simulink model "Mission__SimulatorModel"  (Simulink 10.1)
settings: Solver=ode8  StartTime=0.0  StopTime=100000  FixedStep=time_step  RelTol=1e-3
StartFcn:
  | % copyfile(char(CurrentFolder + "\3DModels\" + string(MODELO_3D)), char(CurrentFolder + "\" + string(MODELO_3D)));
StopFcn:
  | % delete(MODELO_3D)
values from neighbouring files (symbols this model uses):
  Aileron_Trim = -deltaa_trim_med/2    [Trim_ArcDME2.m]
  Elevator_Trim = deltae_trim_med    [Trim_ArcDME2.m]    (also in Trim_ClimbXZ2.m; Trim_CruiseThetaXZ2.m)
  Engine_Trim = lever_trim_med    [Trim_ArcDME2.m]    (also in Trim_ClimbXZ2.m; Trim_CruiseThetaXZ2.m)
  phi_ini = phi_ini_trim_med    [Trim_ArcDME2.m]
  u_ini = u_ini_trim_med    [Trim_ArcDME2.m]    (also in Trim_ClimbXZ2.m; Trim_CruiseThetaXZ2.m)
  v_ini = v_ini_trim2    [Trim_ArcDME2.m]    (also in Trim_ClimbXZ2.m; Trim_CruiseThetaXZ2.m)
  w_ini = -UVW_aux(3)    [Trim_ArcDME2.m]    (also in Trim_ClimbXZ2.m = -UVW_aux2(3) + UVW_aux1(3); Trim_CruiseThetaXZ2.m)
undefined symbols (not defined in the file or in its folder): AoA_alpha_max, AoA_beta_max, b, c, cargo_mass, CD0_interp, CD_ajus_coef, CD_beta_interp, CD_mach_reg, CDde, CDflap, CDgear, CDi, CDsb, CDsp, CL_ajus_coef, CL_alpha_interp, CL_alpha_reg, Clb, Clda_interp, CLde, Cldr, Clp, Clr, Cm0, Cm_alpha, Cmadot, Cmde_ajus_coef, Cmde_interp, Cmq, Cnb, Cndr, Cnr, Coef_Aileron_Beta, Coef_Aileron_Phi, Coef_Aileron_Rudder, Coef_Elevator_Alpha, Coef_Rudder_Aileron, Coef_Rudder_Beta, CYb, dCLflap, dfuel, dfuel0, e0_0, e1_0, e2_0, e3_0, fuel, fuel_density, fuel_max, g, GeoDate_Ap, GeoDate_Day, GeoDate_LatLongElv, GeoDate_Time, Ixx, Ixz, Iyy, Izz, kCDge_interp ... (+35)
libraries: aerolibconvert2 x17, aerolibutil x14, dsppolyfun x7, aerolibactuator x5, sharedtransform x4, robotcorelib x4, simulink x3, visionstatistics x3, vrlib x2, aerolibasang x1
(part 3 of 3)

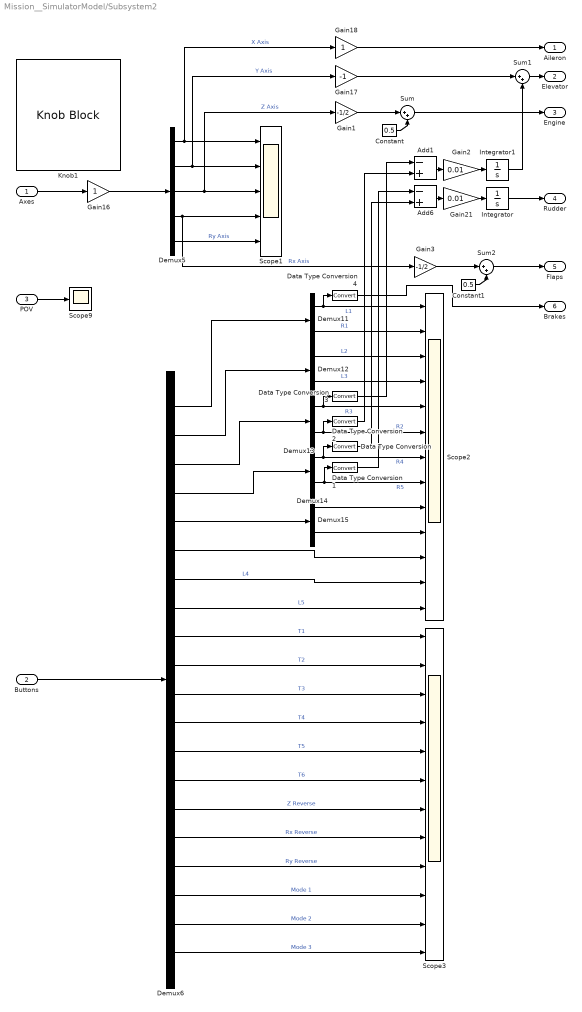
== system Mission__SimulatorModel/Subsystem2 ==
  Axes : Inport
  Buttons : Inport  Port=2
  POV : Inport  Port=3
  Add1 : Sum  Inputs=-+
  Add6 : Sum  Inputs=-+
  Constant : Constant  Value=0.5
  Constant1 : Constant  Value=0.5
  Data Type Conversion{,1..4} (5 alike) : DataTypeConversion
  Demux{11..15} (5 alike) : Demux  Outputs=2
  Demux5 : Demux  Outputs=5
  Demux6 : Demux  Outputs=20
  Gain1 : Gain  Gain=-1/2
  Gain16 : Gain
  Gain17 : Gain  Gain=-1
  Gain18 : Gain
  Gain2 : Gain  Gain=0.01
  Gain21 : Gain  Gain=0.01
  Gain3 : Gain  Gain=-1/2
  Integrator : Integrator  LowerSaturationLimit=inf
  Integrator1 : Integrator  LowerSaturationLimit=inf
  Knob1 : KnobBlock  LabelPosition=Hide  ScaleMax=1
  Scope1 : Scope  NumInputPorts=5
  Scope2 : Scope  NumInputPorts=13
  Scope3 : Scope  NumInputPorts=12
  Scope9 : Scope
  Sum : Sum  Inputs=|++
  Sum1 : Sum  Inputs=|++
  Sum2 : Sum  Inputs=|++
  Aileron : Outport
  Elevator : Outport  Port=2
  Engine : Outport  Port=3
  Rudder : Outport  Port=4
  Flaps : Outport  Port=5
  Brakes : Outport  Port=6
  wires:
  Demux5/1 -> Gain18/1, Scope1/1  "X Axis"
  Demux6/8 -> Scope2/13  "L5"
  Demux6/12 -> Scope3/4  "T4"
  Add6/1 -> Gain21/1
  Data Type Conversion1/1 -> Add6/1
  Demux6/14 -> Scope3/6  "T6"
  Demux12/2 -> Scope2/4  "L3"
  Demux6/10 -> Scope3/2  "T2"
  Buttons/1 -> Demux6/1
  Demux5/3 -> Gain1/1, Scope1/3  "Z Axis"
  Demux5/2 -> Gain17/1, Scope1/2  "Y Axis"
  Demux6/13 -> Scope3/5  "T5"
  POV/1 -> Scope9/1
  Demux15/2 -> Scope2/10
  Demux14/2 -> Data Type Conversion1/1, Scope2/8  "R5"
  Demux6/9 -> Scope3/1  "T1"
  Demux14/1 -> Data Type Conversion/1, Scope2/7  "R4"
  Demux6/18 -> Scope3/10  "Mode 1"
  Demux12/1 -> Scope2/3  "L2"
  Data Type Conversion/1 -> Add6/2
  Gain16/1 -> Demux5/1
  Demux6/17 -> Scope3/9  "Ry Reverse"
  Gain21/1 -> Integrator/1
  Demux6/16 -> Scope3/8  "Rx Reverse"
  Demux11/1 -> Data Type Conversion4/1, Scope2/1  "L1"
  Demux13/1 -> Data Type Conversion3/1, Scope2/5  "R3"
  Demux6/19 -> Scope3/11  "Mode 2"
  Demux5/5 -> Scope1/5  "Ry Axis"
  Demux11/2 -> Scope2/2  "R1"
  Demux6/15 -> Scope3/7  "Z Reverse"
  Demux6/4 -> Demux14/1
  Demux6/6 -> Scope2/11
  Demux6/5 -> Demux15/1
  Demux5/4 -> Gain3/1, Scope1/4  "Rx Axis"
  Demux15/1 -> Scope2/9
  Demux13/2 -> Data Type Conversion2/1, Scope2/6  "R2"
  Axes/1 -> Gain16/1
  Demux6/1 -> Demux11/1
  Demux6/2 -> Demux12/1
  Demux6/3 -> Demux13/1
  Demux6/11 -> Scope3/3  "T3"
  Demux6/7 -> Scope2/12  "L4"
  Demux6/20 -> Scope3/12  "Mode 3"
  Gain18/1 -> Aileron/1
  Integrator/1 -> Rudder/1
  Gain1/1 -> Sum/1
  Constant/1 -> Sum/2
  Sum/1 -> Engine/1
  Gain2/1 -> Integrator1/1
  Add1/1 -> Gain2/1
  Data Type Conversion3/1 -> Add1/1
  Data Type Conversion2/1 -> Add1/2
  Gain17/1 -> Sum1/1
  Sum1/1 -> Elevator/1
  Integrator1/1 -> Sum1/2
  Constant1/1 -> Sum2/2
  Gain3/1 -> Sum2/1
  Sum2/1 -> Flaps/1
  Data Type Conversion4/1 -> Brakes/1

== system Mission__SimulatorModel/Subsystem3 ==
  Altura : Inport
  Mx : Inport  Port=2
  Constant7 : Constant  Value=0
  Switch5 : Switch  Criteria=u2 > Threshold
  Mx con Suelo : Outport
  wires:
  Constant7/1 -> Switch5/3
  Switch5/1 -> Mx con Suelo/1
  Mx/1 -> Switch5/1
  Altura/1 -> Switch5/2

== system Mission__SimulatorModel/Subsystem4 ==
  Altura : Inport
  Mz : Inport  Port=2
  Constant7 : Constant  Value=0
  Switch5 : Switch  Criteria=u2 > Threshold
  Mz con Suelo : Outport
  wires:
  Altura/1 -> Switch5/2
  Mz/1 -> Switch5/1
  Switch5/1 -> Mz con Suelo/1
  Constant7/1 -> Switch5/3

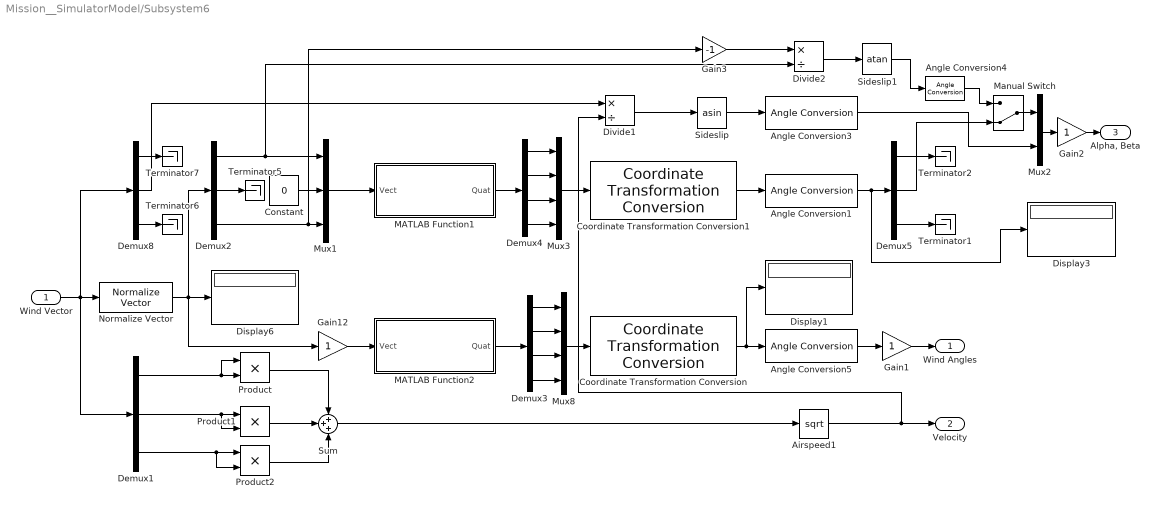
== system Mission__SimulatorModel/Subsystem6 ==
  Wind Vector : Inport
  Airspeed1 : Sqrt  AlgorithmType=Newton-Raphson  SaturateOnIntegerOverflow=on
  Angle Conversion{1,3..5} (4 alike) : aerolibconvert2/Angle Conversion  IU=rad  OU=deg
  Constant : Constant  Value=0
  Coordinate Transformation Conversion : robotcorelib/Coordinate Transformation Conversion  InputRepresentation=Quaternion  InputEulerSequence=ZYX  ShowTrVecInputPort=on  OutputRepresentation=Euler Angles  OutputEulerSequence=XYZ  ShowTrVecOutputPort=on  SimulateUsing=Interpreted execution
      settings: SourceProductBaseCode=NV,RO,RR
  Coordinate Transformation Conversion1 : robotcorelib/Coordinate Transformation Conversion  InputRepresentation=Quaternion  InputEulerSequence=ZYX  ShowTrVecInputPort=on  OutputRepresentation=Euler Angles  OutputEulerSequence=XYZ  ShowTrVecOutputPort=on  SimulateUsing=Interpreted execution
      settings: SourceProductBaseCode=NV,RO,RR
  Demux{1..2,5,8} (4 alike) : Demux  Outputs=3
  Demux3 : Demux
  Demux4 : Demux
  Display1 : Display
  Display3 : Display
  Display6 : Display
  Divide1 : Product  Inputs=*/
  Divide2 : Product  Inputs=*/
  Gain1 : Gain
  Gain12 : Gain
  Gain2 : Gain
  Gain3 : Gain  Gain=-1
  MATLAB Function1 : MATLAB Function  TreatAsAtomicUnit=on
  MATLAB Function2 : MATLAB Function  TreatAsAtomicUnit=on
  Manual Switch : ManualSwitch  CurrentSetting=0
  Mux1 : Mux  Inputs=3
  Mux2 : Mux  Inputs=2
  Mux3 : Mux
  Mux8 : Mux
  Normalize Vector : vrlib/Utilities/Normalize Vector  maxzero=0
  Product : Product  RndMeth=Zero
  Product1 : Product  RndMeth=Zero
  Product2 : Product  RndMeth=Zero
  Sideslip : Trigonometry  Operator=asin
  Sideslip1 : Trigonometry  Operator=atan
  Sum : Sum  Inputs=+++
  Terminator{1..2,5..7} (5 alike) : Terminator
  Wind Angles : Outport
  Velocity : Outport  Port=2  InitialOutput=0  VectorParamsAs1DForOutWhenUnconnected=off
  "Alpha, Beta" : Outport  Port=3  InitialOutput=0  VectorParamsAs1DForOutWhenUnconnected=off
  wires:
  Gain1/1 -> Wind Angles/1
  Airspeed1/1 -> Divide1/2, Velocity/1
  Product1/1 -> Sum/2
  Demux1/1 -> Product/2, Product/1
  Sum/1 -> Airspeed1/1
  Demux1/3 -> Product2/2, Product2/1
  Product/1 -> Sum/1
  Product2/1 -> Sum/3
  Demux1/2 -> Product1/1, Product1/2
  MATLAB Function2/1(Quat) -> Demux3/1
  Mux8/1 -> Coordinate Transformation Conversion/1
  Demux3/3 -> Mux8/3
  Gain12/1 -> MATLAB Function2/1(Vect)
  Coordinate Transformation Conversion/1 -> Angle Conversion5/1, Display1/1
  Demux3/2 -> Mux8/2
  Wind Vector/1 -> Demux8/1, Normalize Vector/1, Demux1/1
  Angle Conversion5/1 -> Gain1/1
  Demux3/1 -> Mux8/1
  Normalize Vector/1 -> Demux2/1, Display6/1, Gain12/1
  Demux3/4 -> Mux8/4
  Constant/1 -> Mux1/2
  Demux2/1 -> Divide2/2, Mux1/1
  Demux4/4 -> Mux3/4
  Coordinate Transformation Conversion1/1 -> Angle Conversion1/1
  Demux4/3 -> Mux3/3
  Mux3/1 -> Coordinate Transformation Conversion1/1
  Mux1/1 -> MATLAB Function1/1(Vect)
  Demux4/2 -> Mux3/2
  Demux4/1 -> Mux3/1
  Demux2/3 -> Gain3/1, Mux1/3
  MATLAB Function1/1(Quat) -> Demux4/1
  Angle Conversion1/1 -> Display3/1, Demux5/1
  Demux5/3 -> Terminator1/1
  Demux5/1 -> Terminator2/1
  Gain2/1 -> "Alpha, Beta"/1
  Mux2/1 -> Gain2/1
  Sideslip/1 -> Angle Conversion3/1
  Divide1/1 -> Sideslip/1
  Demux8/2 -> Divide1/1
  Demux2/2 -> Terminator5/1
  Demux8/3 -> Terminator6/1
  Demux8/1 -> Terminator7/1
  Angle Conversion3/1 -> Mux2/2
  Manual Switch/1 -> Mux2/1
  Demux5/2 -> Manual Switch/2
  Divide2/1 -> Sideslip1/1
  Angle Conversion4/1 -> Manual Switch/1
  Sideslip1/1 -> Angle Conversion4/1
  Gain3/1 -> Divide2/1

== system Mission__SimulatorModel/Subsystem9 ==
  Initial Mass : Inport
  Fuel : Inport  Port=2
  Cargo : Inport  Port=3
  Engine : Inport  Port=4
  "       " : Constant  Value=dfuel0
  "          " : Constant  Value=fuel_max * fuel_density
  "              " : Constant  Value=0
  "                  " : Constant  Value=dfuel
  Abs : Abs
  Add : Sum  Inputs=+++-
  Add1 : Sum  Inputs=+-
  Display : Display
  Divide : Product  Inputs=/*
  Gain1 : Gain  Gain=100
  Gain2 : Gain  Gain=fuel_density
  Gain3 : Gain  Gain=NMotores
  Gain4 : Gain  Gain=NMotores
  Integrator : Integrator  InitialConditionSource=external
  Product : Product
  Saturation : Saturate  UpperLimit=1  LowerLimit=0
  Saturation Dynamic : simulink/Discontinuities/Saturation Dynamic  OutMin=[]  OutMax=[]  OutDataTypeStr=Inherit: Same as second input  OutDataType=fixdt(1, 16)  OutScaling=2^-10  DoSatur=off
  Real Mass : Outport
  Fuel Capacity : Outport  Port=2
  Fuel Flow [kg/s] : Outport  Port=3
  wires:
  Initial Mass/1 -> Add/1
  Fuel/1 -> Gain2/1
  Cargo/1 -> Add/3
  Engine/1 -> Abs/1
  "       "/1 -> Gain4/1
  Abs/1 -> Product/2
  "                  "/1 -> Gain3/1
  Product/1 -> Fuel Flow [kg/s]/1, Integrator/1
  Add/1 -> Real Mass/1
  Add1/1 -> Divide/2
  Divide/1 -> Saturation/1, Gain1/1
  Gain1/1 -> Display/1
  Integrator/1 -> Saturation Dynamic/2
  Saturation Dynamic/1 -> Add1/2, Add/4
  "              "/1 -> Saturation Dynamic/3
  Gain2/1 -> Saturation Dynamic/1, Add1/1, Add/2
  Saturation/1 -> Fuel Capacity/1
  "          "/1 -> Divide/1
  Gain3/1 -> Product/1
  Gain4/1 -> Integrator/2

== system Mission__SimulatorModel/6DOF (Ejes Cuerpo)/Subsystem ==
  p q r : Inport
  q0 q1 q2 q3 : Inport  Port=2
  Constant : Constant
  Dot Product : DotProduct  OutDataTypeStr=Inherit: Inherit via internal rule
  Mux1 : Mux  Inputs=[3 4 1]
  Mux2 : Mux
  Sum : Sum  Inputs=|+-  InputSameDT=on  SaturateOnIntegerOverflow=on  OutDataTypeStr=Inherit: Same as first input
  q0dot : Fcn  Expr=-0.5 * ( u[5]*u[1]+u[6]*u[2]+u[7]*u[3] ) + u[8]*u[4]
  q1dot : Fcn  Expr=0.5 * ( u[4]*u[1]+u[6]*u[3]-u[7]*u[2] ) + u[8]*u[5]
  q2dot : Fcn  Expr=0.5 * ( u[4]*u[2]+u[7]*u[1]-u[5]*u[3] ) + u[8]*u[6]
  q3dot : Fcn  Expr=0.5 * ( u[4]*u[3]+u[5]*u[2]-u[6]*u[1] ) + u[8]*u[7]
  qdot : Outport  InitialOutput=0  VectorParamsAs1DForOutWhenUnconnected=off
  wires:
  q0dot/1 -> Mux2/1
  p q r/1 -> Mux1/1
  Dot Product/1 -> Sum/2
  Mux1/1 -> q1dot/1, q0dot/1, q3dot/1, q2dot/1
  Constant/1 -> Sum/1
  q0 q1 q2 q3/1 -> Mux1/2, Dot Product/2, Dot Product/1
  Mux2/1 -> qdot/1
  Sum/1 -> Mux1/3
  q3dot/1 -> Mux2/4
  q1dot/1 -> Mux2/2
  q2dot/1 -> Mux2/3

== system Mission__SimulatorModel/Fuerzas Aerodinamicas/Subsystem qS ==
  rho : Inport
  S : Inport  Port=2
  V : Inport  Port=3
  Gain : Gain  Gain=0.5
  Math Function : Math  Operator=square  SaturateOnIntegerOverflow=on
  Product : Product
  Product1 : Product
  qS : Outport
  wires:
  Product/1 -> Product1/1
  rho/1 -> Product/1
  Gain/1 -> Product/2
  Math Function/1 -> Gain/1
  S/1 -> Product1/2
  V/1 -> Math Function/1
  Product1/1 -> qS/1  "qS"

== system Mission__SimulatorModel/Subsystem15/Jump Limiter ==
  "Input " : Inport
  Constant6 : Constant
  Delay3 : Delay  InitialCondition=0
  Sum1 : Sum  Inputs=|+-
  Sum2 : Sum  Inputs=|+-
  Sum3 : Sum  Inputs=|+-
  Switch3 : Switch  Criteria=u2 > Threshold  Threshold=1
  Output Limited : Outport
  wires:
  "Input "/1 -> Switch3/3, Sum3/1, Sum1/1, Delay3/1
  Sum3/1 -> Switch3/1
  Constant6/1 -> Sum2/2
  Sum1/1 -> Sum2/1, Switch3/2
  Switch3/1 -> Output Limited/1
  Sum2/1 -> Sum3/2
  Delay3/1 -> Sum1/2

== system Mission__SimulatorModel/Subsystem15/Signal Restarter ==
  Full Signal : Inport
  Index : Inport  Port=2
  Abs : Abs
  Delay2 : Delay  DelayLength=4  InitialCondition=0
  Delay3 : Delay  DelayLength=1  InitialCondition=0
  Derivative : Derivative
  Gain : Gain  Gain=1000000000
  Integrator : Integrator  LimitOutput=on  LowerSaturationLimit=0
  Memory : Memory
  Sum1 : Sum  Inputs=|+-
  Sum2 : Sum  Inputs=|+-
  Switch : Switch  Criteria=u2 ~= 0  Threshold=5
  Zero-Order Hold : ZeroOrderHold  SampleTime=-1
  Trunked Signal : Outport
  wires:
  Abs/1 -> Memory/1
  Index/1 -> Sum2/2, Delay3/1
  Sum2/1 -> Switch/2
  Switch/1 -> Integrator/1, Abs/1
  Delay3/1 -> Sum2/1
  Derivative/1 -> Switch/3, Sum1/1
  Delay2/1 -> Sum1/2
  Sum1/1 -> Switch/1
  Memory/1 -> Gain/1
  Gain/1 -> Zero-Order Hold/1
  Zero-Order Hold/1 -> Delay2/1
  Full Signal/1 -> Derivative/1
  Integrator/1 -> Trunked Signal/1

== system Mission__SimulatorModel/Subsystem16/Subsystem15 ==
  Lat_Long_h : Inport
  X : Inport  Port=2
  Y : Inport  Port=3
  h : Inport  Port=4
  Data Type Conversion : DataTypeConversion  RndMeth=Nearest
  Data Type Conversion1 : DataTypeConversion  RndMeth=Nearest
  Data Type Conversion2 : DataTypeConversion  RndMeth=Nearest
  MATLAB Function : MATLAB Function  TreatAsAtomicUnit=on
  MATLAB Function1 : MATLAB Function  TreatAsAtomicUnit=on
  Mux : Mux  Inputs=3
  Saturation : Saturate  UpperLimit=inf  LowerLimit=0
  Sum3 : Sum  Inputs=++|
  Sum4 : Sum  Inputs=++|
  Sum5 : Sum  Inputs=|++
  New Lat_Long_h : Outport
  wires:
  Data Type Conversion/1 -> Sum3/1
  Mux/1 -> New Lat_Long_h/1
  Data Type Conversion1/1 -> Sum4/1
  MATLAB Function/2(Y_UTM) -> Sum4/2
  MATLAB Function/4(h) -> Sum5/1
  Sum5/1 -> Saturation/1
  Sum4/1 -> MATLAB Function1/2(Y_UTM)
  Data Type Conversion2/1 -> Sum5/2
  Sum3/1 -> MATLAB Function1/1(X_UTM)
  MATLAB Function/1(X_UTM) -> Sum3/2
  MATLAB Function1/2(Lon) -> Mux/2
  MATLAB Function1/1(Lat) -> Mux/1
  MATLAB Function1/3(h) -> Mux/3
  MATLAB Function/3(Zone_UTM) -> MATLAB Function1/3(Zone_UTM)
  Lat_Long_h/1 -> MATLAB Function/1(Lat_Long_h)
  Y/1 -> Data Type Conversion1/1
  X/1 -> Data Type Conversion/1
  h/1 -> Data Type Conversion2/1
  Saturation/1 -> MATLAB Function1/4("h ")

== system Mission__SimulatorModel/Subsystem17/Propulsión en función de las  condiciones de Vuelo ==
  Mach : Inport
  h : Inport  Port=2
  Traccion : Inport  Port=3
  MATLAB Function1 : MATLAB Function  TreatAsAtomicUnit=on
  Traccion por Motor1 : Constant  Value=KT
  Traccion por Motor2 : Constant  Value=KT_mach
  Traccion por Motor3 : Constant  Value=KT_rho
  Trac : Outport
  wires:
  Traccion/1 -> MATLAB Function1/3(Traccion)
  Traccion por Motor1/1 -> MATLAB Function1/4(KT)
  Traccion por Motor3/1 -> MATLAB Function1/5(KT_rho)
  Traccion por Motor2/1 -> MATLAB Function1/6(KT_mach)
  h/1 -> MATLAB Function1/2(h)
  Mach/1 -> MATLAB Function1/1(Mach)
  MATLAB Function1/1(Trac) -> Trac/1

== matlab function Subsystem6/MATLAB Function2 ==
  data: Vect input double; Quat output double
function Quat = Vector_to_Quaternion(Vect)
v1 = [1 0 0]
v2 = Vect


a = cross(v1, v2);
xyz = a;
w = sqrt((norm(v1) ^ 2) * (norm(v2) ^ 2)) + dot(v1, v2);

aux = v1(1)*v2(1);
if aux < 0
    q = [-w,xyz];
else
    q = [w,xyz];
end

Quat = q;

== matlab function Subsystem15/MATLAB Function ==
  data: OpData input double; d1 output double; Index input double; StateData input double; d2 output double; d3 output double; c0 output double; c_alt output double; c_vel output double; c_hdg output double; stop output double; next output double; psi_ini input double
function [d1,d2,d3,c0,c_alt,c_vel,c_hdg,stop,next] = fcn(OpData,Index,StateData,psi_ini)

[m,n] = size(OpData);
if Index > m
        stop = 1;
        Op = 0;
else
    if round(Index) <= 0
        Op = OpData(1,1);
    else
        Op = OpData(round(Index),1);
    end
    
    stop = 0;
end

next = 0;

c0 = 0;
c_alt = 0;
c_vel = 0;
c_hdg = 0;
d1 = 0;
d2 = 0;
d3 = 0;

if Op == 9
    stop = 1;
end

if Op == 0
end

if Op == 1
    d1 = 450;
    d2 = 120;
    d3 = psi_ini*180/pi;
    c_vel = 1;
    c0 = 1;
    
    if StateData(1) >= 60
        c_alt = 1;
        c_hdg = 1;
    end
    
    if StateData(2) >= 140
        c_vel = 0;
        c_alt = 0;
        c_hdg = 0;
        c0 = 0;
%         next = round(Index);
        next = 1;
        
    end
%     if Index > m
%             stop = 1;
%         end
end

if Op == 2
%     if OpData(round(Index)-1,1) == Op
%         next = round(Index)-2;
%     else
%         next = round(Index)-1;
%     end
    if round(Index) == 0
        Index = Index+1;
    end
    d1 = OpData(round(Index),2);
    d2 = OpData(round(Index),3);
    d3 = OpData(round(Index),5);
    c_alt = 1;
    c_vel = 1;
    c_hdg = 1;
    c0 = 1;
    
    if StateData(3) >= OpData(round(Index),4)
        c_vel = 0;
        c_alt = 0;
        c_hdg = 0;
        c0 = 0;
        
%         if OpData(round(Index)-1,1) == Op
%             next = round(Index)-1;
%         else
%         next = round(Index);
%         end
        next = 1;
        
        
    end
%     if Index > m
%             stop = 1;
%         end
end

== matlab function Subsystem16/Subsystem15/MATLAB Function ==
  data: Lat_Long_h input double; X_UTM output double; Y_UTM output double; Zone_UTM output double; h output double
function [X_UTM, Y_UTM, Zone_UTM, h] = fcn(Lat_Long_h)
Lat = Lat_Long_h(1);
Lon = Lat_Long_h(2);
h = Lat_Long_h(3);


    n1=length(Lat);
    n2=length(Lon);
    if (n1~=n2)
       error('Lat and Lon vectors should have the same length');
    end


    % Memory pre-allocation
    
    x=zeros(n1,1);
    y=zeros(n1,1);
    utmzone = zeros(n1,4);utmzone = char(utmzone);
    utmzone(n1,:)='60 X';

       la=Lat;
       lo=Lon;

       sa = 6378137.000000 ; sb = 6356752.314245;

       e2 = ( ( ( sa ^ 2 ) - ( sb ^ 2 ) ) ^ 0.5 ) / sb;
       e2cuadrada = e2 ^ 2;
       c = ( sa ^ 2 ) / sb;


       lat = la * ( pi / 180 );
       lon = lo * ( pi / 180 );

       Huso = fix( ( lo / 6 ) + 31);
       S = ( ( Huso * 6 ) - 183 );
       deltaS = lon - ( S * ( pi / 180 ) );

       if (la<-72), Letra= 1;% 'C';
       elseif (la<-64), Letra= 2;% 'D';
       elseif (la<-56), Letra= 3;% 'E';
       elseif (la<-48), Letra= 4;% 'F';
       elseif (la<-40), Letra= 5;% 'G';
       elseif (la<-32), Letra= 6;% 'H';
       elseif (la<-24), Letra= 7;% 'J';
       elseif (la<-16), Letra= 8;% 'K';
       elseif (la<-8), Letra= 9;% 'L';
       elseif (la<0), Letra= 10;% 'M';
       elseif (la<8), Letra= 11;% 'N';
       elseif (la<16), Letra= 12;% 'P';
       elseif (la<24), Letra= 13;% 'Q';
       elseif (la<32), Letra= 14;% 'R';
       elseif (la<40), Letra= 15;% 'S';
       elseif (la<48), Letra= 16;% 'T';
       elseif (la<56), Letra= 17;% 'U';
       elseif (la<64), Letra= 18;% 'V';
       elseif (la<72), Letra= 19;% 'W';
       else Letra= 20;% 'X';
       end

       a = cos(lat) * sin(deltaS);
       epsilon = 0.5 * log( ( 1 +  a) / ( 1 - a ) );
       nu = atan( tan(lat) / cos(deltaS) ) - lat;
       v = ( c / ( ( 1 + ( e2cuadrada * ( cos(lat) ) ^ 2 ) ) ) ^ 0.5 ) * 0.9996;
       ta = ( e2cuadrada / 2 ) * epsilon ^ 2 * ( cos(lat) ) ^ 2;
       a1 = sin( 2 * lat );
       a2 = a1 * ( cos(lat) ) ^ 2;
       j2 = lat + ( a1 / 2 );
       j4 = ( ( 3 * j2 ) + a2 ) / 4;
       j6 = ( ( 5 * j4 ) + ( a2 * ( cos(lat) ) ^ 2) ) / 3;
       alfa = ( 3 / 4 ) * e2cuadrada;
       beta = ( 5 / 3 ) * alfa ^ 2;
       gama = ( 35 / 27 ) * alfa ^ 3;
       Bm = 0.9996 * c * ( lat - alfa * j2 + beta * j4 - gama * j6 );
       xx = epsilon * v * ( 1 + ( ta / 3 ) ) + 500000;
       yy = nu * v * ( 1 + ta ) + Bm;

       if (yy<0)
           yy=9999999+yy;
       end

       x=xx;
       y=yy;
        utmzone = [Huso Letra];

X_UTM = 0; Y_UTM = 0; 
X_UTM = x; Y_UTM = y; 
Zone_UTM = utmzone;

== matlab function Subsystem17/Propulsión en función de las condiciones de Vuelo/MATLAB Function1 ==
  data: Mach input double; Trac output double; h input double; Traccion input double; KT input double; KT_rho input double; KT_mach input double
function Trac  = Trac(Mach,h,Traccion,KT,KT_rho,KT_mach)

rho = h*3.28084

if rho >= KT_rho(1) && rho <= KT_rho(2)
        aux_rho1 = (rho - KT_rho(1))/(KT_rho(2) - KT_rho(1))
        aux_rho2 = [1,2]

else
    if rho >= KT_rho(2) && rho <= KT_rho(3)
        aux_rho1 = (rho - KT_rho(2))/(KT_rho(3) - KT_rho(2))
        aux_rho2 = [2,3]
    
    else
        if rho >= KT_rho(3) && rho <= KT_rho(4)
        aux_rho1 = (rho - KT_rho(3))/(KT_rho(4) - KT_rho(3))
        aux_rho2 = [3,4]
        
            else
                if rho >= KT_rho(4) && rho <= KT_rho(5)
        aux_rho1 = (rho - KT_rho(4))/(KT_rho(5) - KT_rho(4))
        aux_rho2 = [4,5]

                else
        aux_rho1 = (rho - KT_rho(5))/(KT_rho(8) - KT_rho(5))
        aux_rho2 = [5,8]
        end
    end
    end
end

if Mach >= KT_mach(1) && Mach <= KT_mach(2)
        aux_mach1 = (Mach - KT_mach(1))/(KT_mach(2) - KT_mach(1))
        aux_mach2 = [1,2]

else
    if Mach >= KT_mach(2) && Mach <= KT_mach(3)
        aux_mach1 = (Mach - KT_mach(2))/(KT_mach(3) - KT_mach(2))
        aux_mach2 = [2,3]
    
    else
        if Mach >= KT_mach(3) && Mach <= KT_mach(4)
        aux_mach1 = (Mach - KT_mach(3))/(KT_mach(4) - KT_mach(3))
        aux_mach2 = [3,4]
        
            else
                if Mach >= KT_mach(4) && Mach <= KT_mach(5)
        aux_mach1 = (Mach - KT_mach(4))/(KT_mach(5) - KT_mach(4))
        aux_mach2 = [4,5]

                else if Mach >= KT_mach(5) && Mach <= KT_mach(6)
        aux_mach1 = (Mach - KT_mach(5))/(KT_mach(6) - KT_mach(5))
        aux_mach2 = [5,6]

                    else
        aux_mach1 = (Mach - KT_mach(6))/(KT_mach(7) - KT_mach(6))
        aux_mach2 = [6,7]
                    end
        end
        end
    end
end

k1 = (KT(aux_rho2(2),aux_mach2(1)) - KT(aux_rho2(1),aux_mach2(1)))*aux_rho1 + KT(aux_rho2(1),aux_mach2(1))
k2 = (KT(aux_rho2(2),aux_mach2(2)) - KT(aux_rho2(1),aux_mach2(2)))*aux_rho1 + KT(aux_rho2(1),aux_mach2(2))
k3 = (k2-k1)*aux_mach1 + k1

    Trac = Traccion * k3

== matlab function Subsystem6/MATLAB Function1 ==
  data: Vect input double; Quat output double
function Quat = Vector_to_Quaternion(Vect)
v1 = [1 0 0]
v2 = Vect


a = cross(v1, v2);
xyz = a;
w = sqrt((norm(v1) ^ 2) * (norm(v2) ^ 2)) + dot(v1, v2);

aux = v1(1)*v2(1);
if aux < 0
    q = [-w,xyz];
else
    q = [w,xyz];
end

Quat = q;

== matlab function Fuerzas Aerodinamicas/MATLAB Function2 ==
  data: temp input double; V input double; CD_mach output double; CD_mach_reg input double; Mach output double
function [CD_mach,Mach] = CD_mach(temp,V,CD_mach_reg)

Vs = sqrt(1.4*8.314*temp/0.029)
Mach = V/Vs;


if Mach >= CD_mach_reg(1,1) && Mach <= CD_mach_reg(2,1)
        CD_mach = (CD_mach_reg(2,2)-CD_mach_reg(1,2)) / (CD_mach_reg(2,1)-CD_mach_reg(1,1)) * (Mach-CD_mach_reg(1,1)) + CD_mach_reg(1,2);

else
    if Mach >= CD_mach_reg(2,1) && Mach <= CD_mach_reg(3,1)
        CD_mach = (CD_mach_reg(3,2)-CD_mach_reg(2,2)) / (CD_mach_reg(3,1)-CD_mach_reg(2,1)) * (Mach-CD_mach_reg(2,1)) + CD_mach_reg(2,2);
    
    else
        if Mach >= CD_mach_reg(3,1) && Mach <= CD_mach_reg(4,1)
        CD_mach = (CD_mach_reg(4,2)-CD_mach_reg(3,2)) / (CD_mach_reg(4,1)-CD_mach_reg(3,1)) * (Mach-CD_mach_reg(3,1)) + CD_mach_reg(3,2);
        
            else
                CD_mach = 0
        end
    end
end
end

== matlab function Subsystem16/Subsystem15/MATLAB Function1 ==
  data: X_UTM input double; Lat output double; Y_UTM input double; Zone_UTM input double; h input double; Lon output double; h output double
function [Lat,Lon,h]  = fcn(X_UTM, Y_UTM, Zone_UTM, h)
xx = X_UTM; yy = Y_UTM; utmzone = Zone_UTM;

    n1=length(xx);
    n2=length(yy);




    % Memory pre-allocation
    
    Lat=zeros(n1,1);
    Lon=zeros(n1,1);



       if (utmzone(2)>20 || utmzone(2)<1) %if (utmzone(i,4)>'X' || utmzone(i,4)<'C')
       end
       if (utmzone(2)>10)
          hemis='N';   % Northern hemisphere
       else
          hemis='S';
       end

       x=xx;
       y=yy;
       zone=utmzone(1);

       sa = 6378137.000000 ; sb = 6356752.314245;

       e2 = ( ( ( sa ^ 2 ) - ( sb ^ 2 ) ) ^ 0.5 ) / sb;
       e2cuadrada = e2 ^ 2;
       c = ( sa ^ 2 ) / sb;

       X = x - 500000;

       if hemis == 'S' || hemis == 's'
           Y = y - 10000000;
       else
           Y = y;
       end

       S = ( ( zone * 6 ) - 183 ); 
       lat =  Y / ( 6366197.724 * 0.9996 );                                    
       v = ( c / ( ( 1 + ( e2cuadrada * ( cos(lat) ) ^ 2 ) ) ) ^ 0.5 ) * 0.9996;
       a = X / v;
       a1 = sin( 2 * lat );
       a2 = a1 * ( cos(lat) ) ^ 2;
       j2 = lat + ( a1 / 2 );
       j4 = ( ( 3 * j2 ) + a2 ) / 4;
       j6 = ( ( 5 * j4 ) + ( a2 * ( cos(lat) ) ^ 2) ) / 3;
       alfa = ( 3 / 4 ) * e2cuadrada;
       beta = ( 5 / 3 ) * alfa ^ 2;
       gama = ( 35 / 27 ) * alfa ^ 3;
       Bm = 0.9996 * c * ( lat - alfa * j2 + beta * j4 - gama * j6 );
       b = ( Y - Bm ) / v;
       Epsi = ( ( e2cuadrada * a^ 2 ) / 2 ) * ( cos(lat) )^ 2;
       Eps = a * ( 1 - ( Epsi / 3 ) );
       nab = ( b * ( 1 - Epsi ) ) + lat;
       senoheps = ( exp(Eps) - exp(-Eps) ) / 2;
       Delt = atan(senoheps / (cos(nab) ) );
       TaO = atan(cos(Delt) * tan(nab));
       longitude = (Delt *(180 / pi ) ) + S;
       latitude = ( lat + ( 1 + e2cuadrada* (cos(lat)^ 2) - ( 3 / 2 ) * e2cuadrada * sin(lat) * cos(lat) * ( TaO - lat ) ) * ( TaO - lat ) ) * ...
                        (180 / pi);

       Lat=(latitude);
       Lon=(longitude);
